simulink library "LossSim_Library"  (Simulink 7.4)
settings: Solver=ode45  StartTime=0.0  StopTime=10.0  RelTol=1e-3
undefined symbols (not defined in the file or in its folder): Ts
settings Model: Creator=CHSAPET  LastModifiedBy=CHSAPET

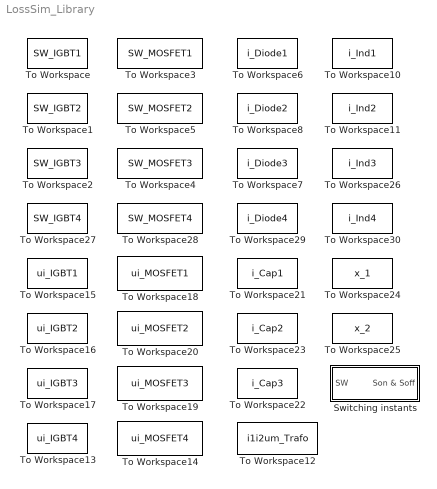
== system LossSim_Library ==
  Switching instants : Subsystem
  To Workspace : ToWorkspace  VariableName=SW_IGBT1  SampleTime=Ts  SaveFormat=Array
      settings: MaxDataPoints=NOS
  To Workspace1 : ToWorkspace  VariableName=SW_IGBT2  SampleTime=Ts  SaveFormat=Array
      settings: MaxDataPoints=NOS
  To Workspace10 : ToWorkspace  VariableName=i_Ind1  SampleTime=Ts  SaveFormat=Array
      settings: MaxDataPoints=NOS
  To Workspace11 : ToWorkspace  VariableName=i_Ind2  SampleTime=Ts  SaveFormat=Array
      settings: MaxDataPoints=NOS
  To Workspace12 : ToWorkspace  VariableName=i1i2um_Trafo  SampleTime=Ts  SaveFormat=Array
      settings: MaxDataPoints=NOS
  To Workspace13 : ToWorkspace  VariableName=ui_IGBT4  SampleTime=Ts  SaveFormat=Array
      settings: MaxDataPoints=NOS
  To Workspace14 : ToWorkspace  VariableName=ui_MOSFET4  SampleTime=Ts  SaveFormat=Array
      settings: MaxDataPoints=NOS
  To Workspace15 : ToWorkspace  VariableName=ui_IGBT1  SampleTime=Ts  SaveFormat=Array
      settings: MaxDataPoints=NOS
  To Workspace16 : ToWorkspace  VariableName=ui_IGBT2  SampleTime=Ts  SaveFormat=Array
      settings: MaxDataPoints=NOS
  To Workspace17 : ToWorkspace  VariableName=ui_IGBT3  SampleTime=Ts  SaveFormat=Array
      settings: MaxDataPoints=NOS
  To Workspace18 : ToWorkspace  VariableName=ui_MOSFET1  SampleTime=Ts  SaveFormat=Array
      settings: MaxDataPoints=NOS
  To Workspace19 : ToWorkspace  VariableName=ui_MOSFET3  SampleTime=Ts  SaveFormat=Array
      settings: MaxDataPoints=NOS
  To Workspace2 : ToWorkspace  VariableName=SW_IGBT3  SampleTime=Ts  SaveFormat=Array
      settings: MaxDataPoints=NOS
  To Workspace20 : ToWorkspace  VariableName=ui_MOSFET2  SampleTime=Ts  SaveFormat=Array
      settings: MaxDataPoints=NOS
  To Workspace21 : ToWorkspace  VariableName=i_Cap1  SampleTime=Ts  SaveFormat=Array
      settings: MaxDataPoints=NOS
  To Workspace22 : ToWorkspace  VariableName=i_Cap3  SampleTime=Ts  SaveFormat=Array
      settings: MaxDataPoints=NOS
  To Workspace23 : ToWorkspace  VariableName=i_Cap2  SampleTime=Ts  SaveFormat=Array
      settings: MaxDataPoints=NOS
  To Workspace24 : ToWorkspace  VariableName=x_1  SampleTime=Ts  SaveFormat=Array
      settings: MaxDataPoints=NOS
  To Workspace25 : ToWorkspace  VariableName=x_2  SampleTime=Ts  SaveFormat=Array
      settings: MaxDataPoints=NOS
  To Workspace26 : ToWorkspace  VariableName=i_Ind3  SampleTime=Ts  SaveFormat=Array
      settings: MaxDataPoints=NOS
  To Workspace27 : ToWorkspace  VariableName=SW_IGBT4  SampleTime=Ts  SaveFormat=Array
      settings: MaxDataPoints=NOS
  To Workspace28 : ToWorkspace  VariableName=SW_MOSFET4  SampleTime=Ts  SaveFormat=Array
      settings: MaxDataPoints=NOS
  To Workspace29 : ToWorkspace  VariableName=i_Diode4  SampleTime=Ts  SaveFormat=Array
      settings: MaxDataPoints=NOS
  To Workspace3 : ToWorkspace  VariableName=SW_MOSFET1  SampleTime=Ts  SaveFormat=Array
      settings: MaxDataPoints=NOS
  To Workspace30 : ToWorkspace  VariableName=i_Ind4  SampleTime=Ts  SaveFormat=Array
      settings: MaxDataPoints=NOS
  To Workspace4 : ToWorkspace  VariableName=SW_MOSFET3  SampleTime=Ts  SaveFormat=Array
      settings: MaxDataPoints=NOS
  To Workspace5 : ToWorkspace  VariableName=SW_MOSFET2  SampleTime=Ts  SaveFormat=Array
      settings: MaxDataPoints=NOS
  To Workspace6 : ToWorkspace  VariableName=i_Diode1  SampleTime=Ts  SaveFormat=Array
      settings: MaxDataPoints=NOS
  To Workspace7 : ToWorkspace  VariableName=i_Diode3  SampleTime=Ts  SaveFormat=Array
      settings: MaxDataPoints=NOS
  To Workspace8 : ToWorkspace  VariableName=i_Diode2  SampleTime=Ts  SaveFormat=Array
      settings: MaxDataPoints=NOS

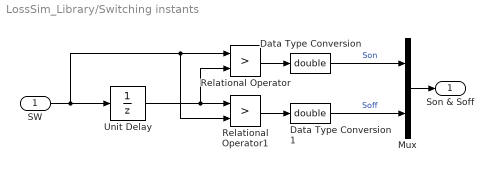
== system LossSim_Library/Switching instants ==
  SW : Inport
  Data Type Conversion : DataTypeConversion  OutDataTypeMode=double  OutDataType=sfix(16)  OutScaling=2^0  OutDataTypeStr=double
  Data Type Conversion1 : DataTypeConversion  OutDataTypeMode=double  OutDataType=sfix(16)  OutScaling=2^0  OutDataTypeStr=double
  Mux : Mux  Inputs=2
  Relational Operator : RelationalOperator  Operator=>  LogicOutDataTypeMode=boolean  OutDataTypeStr=boolean
  Relational Operator1 : RelationalOperator  Operator=>  LogicOutDataTypeMode=boolean  OutDataTypeStr=boolean
  Unit Delay : UnitDelay  SampleTime=Ts
  Son & Soff : Outport
  wires:
  Unit Delay/1 -> Relational Operator/2, Relational Operator1/1
  Relational Operator/1 -> Data Type Conversion/1
  Relational Operator1/1 -> Data Type Conversion1/1
  Data Type Conversion/1 -> Mux/1  "Son"
  Data Type Conversion1/1 -> Mux/2  "Soff"
  SW/1 -> Unit Delay/1, Relational Operator/1, Relational Operator1/2
  Mux/1 -> Son & Soff/1
